simulink model "gm_uz_endat_interface_2023a"  (R2023a)
settings: Solver=FixedStepDiscrete  StartTime=0.0  StopTime=1.3e-3  RelTol=1e-3
undefined symbols (not defined in the file or in its folder): binary_or_gray, bit_sum, delay_first_clk_on_off, endat_clk_divider, endat_encoder_bit_width_multi_turn, endat_encoder_bit_width_single_turn, endat_encoder_number_of_CRC_bits, f_ADC, f_clock, PLL, t_ADC, t_clock
libraries: hdlmdlgenlib x127, simulink x35, hdlsllib x24, simulink_extras x12
(part 3 of 4)

== system gm_uz_endat_interface_2023a/uz_endat_interface/serial_communication/sample_serial_endat_data ==
  note: sample at falling edges of clk
  note: bitset and bit clear
  endat_clk : Inport  OutDataTypeStr=boolean  PortDimensions=1  SampleTime=1e-08
  endat_data : Inport  Port=2  OutDataTypeStr=boolean  PortDimensions=1  SampleTime=1e-08
  sampling_delay_clk_ticks : Inport  Port=3  OutDataTypeStr=uint32  PortDimensions=1  SampleTime=1e-08
  position_sampling_condition_valid : Inport  Port=4  OutDataTypeStr=boolean  PortDimensions=1  SampleTime=1e-08
  Bitwise OR : simulink/Logic and Bit Operations/Bitwise Operator  logicop=OR  UseBitMask=off  NumInputPorts=2  BitMask=double(0)  BitMaskRealWorld=Real World Value
  Bitwise Operator : simulink/Logic and Bit Operations/Bitwise Operator  logicop=AND  UseBitMask=off  NumInputPorts=2  BitMask=double(0)  BitMaskRealWorld=Real World Value
  Bitwise Operator1 : simulink/Logic and Bit Operations/Bitwise Operator  logicop=NOT  UseBitMask=off  BitMask=double(0)  BitMaskRealWorld=Real World Value
  Constant : Constant  Value=0  OutDataTypeStr=boolean  SampleTime=1e-08
  Constant2 : Constant  Value="fi(0,0,64,0,\"hex\",\"0000000000000001\")"  OutDataTypeStr=fixdt(0, 64, 0)  SampleTime=1e-08
  Constant3 : Constant  OutDataTypeStr=boolean  SampleTime=1e-08
  Constant4 : Constant  Value="fi(0,0,64,0,\"hex\",\"0000000000000000\")"  OutDataTypeStr=fixdt(0, 64, 0)  SampleTime=1e-08
  Delay : Delay  DelayLength=double(1)  InitialCondition=0  SampleTime=1e-08
  Delay2 : Delay  DelayLength=double(1)  InitialCondition=0  SampleTime=1e-08
  Detect Rise Positive1 : simulink/Logic and Bit Operations/Detect Rise Positive  vinit=0  OutDataTypeStr=boolean
  Detect Rise Positive2 : simulink/Logic and Bit Operations/Detect Rise Positive  vinit=0  OutDataTypeStr=boolean
  HDL Counter1 : hdlsllib/Sources/HDL Counter  CountType=Free running  CountInit=0  CountStep=1  CountMax=0  CountFromType=Initial value  CountFrom=0  CountResetPort=on  CountLoadPort=off  CountEnbPort=on  CountDirPort=off  CountHitOutputPort=off  CountDataType=Unsigned  CountWordLen=6  CountFracLen=0  CountSampTime=1
  NOT : Logic  Operator=NOT  Inputs=1  AllPortsSameDT=off  OutDataTypeStr=boolean  SampleTime=1e-08
  Relational Operator1 : RelationalOperator  Operator===  OutDataTypeStr=boolean  SampleTime=1e-08  InputSameDT=off
  Relational Operator2 : RelationalOperator  Operator===  OutDataTypeStr=boolean  SampleTime=1e-08  InputSameDT=off
  Sample and Hold1 : Subsystem  mask(Sample and Hold){ic=double(0), Ts=double(1e-08)}
      mask prompts: ic "Initial condition:"; Ts "Sample time:"
      mask help:
      | Sample and hold input signal.
      |
      | The output follows input 1 (In) as long as input 2 (S) is TRUE (1). The output is held when input 2 becomes FALSE (0).
      mask init:
      | Ts = double(1e-08);
      | WantBlockChoice = 'Discrete';
      | block = 'uz_endat_interface_2023a/uz_endat_interface/serial_communication/sample_serial_endat_data/Sample and\nHold1';
      | ic = double(0);
      mask Help: helpview(psbhelp);
      mask Display: disp('S/H')
  Switch : Switch  Criteria=u2 > Threshold  Threshold=double(0)  OutDataTypeStr=boolean  SampleTime=1e-08  SaturateOnIntegerOverflow=off  InputSameDT=off
  Switch1 : Switch  Criteria=u2 > Threshold  Threshold=double(0)  OutDataTypeStr=fixdt(0, 64, 0)  SampleTime=1e-08  SaturateOnIntegerOverflow=off  InputSameDT=off
  Switch3 : Switch  Criteria=u2 > Threshold  Threshold=double(0)  OutDataTypeStr=fixdt(0, 64, 0)  SampleTime=1e-08  SaturateOnIntegerOverflow=off  InputSameDT=off
  Variable Integer Delay : simulink/Discrete/Tapped Delay  vinit=0  samptime=-1  NumDelays=double(100)  DelayOrder=Newest  includeCurrent=on
  multiportswitch : MultiPortSwitch  DataPortOrder=Zero-based contiguous  Inputs=1  DiagnosticForDefault=None  zeroidx=on  SampleTime=1e-08  SaturateOnIntegerOverflow=off  InputSameDT=off
  saturate : Saturate  UpperLimit=double(100)  LowerLimit=double(0)  SampleTime=1e-08  OutDataTypeStr=uint32
  shift arithmetic : ArithShift  BitShiftNumberSource=Input port  BitShiftDirection=Left
      settings: InputPortMap=u0,p1
  endat_data_raw : Outport  OutDataTypeStr=uint64  SampleTime=1e-08
  endat_data_SH : Outport  Port=2  SampleTime=1e-08
  wires:
  Bitwise Operator1/1 -> Bitwise Operator/1
  Constant/1 -> Switch/3
  Constant2/1 -> shift arithmetic/1
  Constant3/1 -> Relational Operator1/2
  Constant4/1 -> Relational Operator2/2
  Detect Rise Positive1/1 -> HDL Counter1/1
  Detect Rise Positive2/1 -> Switch/1
  HDL Counter1/1 -> shift arithmetic/2, Relational Operator2/1
  NOT/1 -> Detect Rise Positive2/1
  Relational Operator1/1 -> Switch1/2
  Relational Operator2/1 -> Switch3/2
  Sample and Hold1/1("   ") -> Relational Operator1/1, endat_data_SH/1
  shift arithmetic/1 -> Bitwise Operator1/1, Bitwise OR/1
  Switch/1 -> Variable Integer Delay/1
  Switch1/1 -> Delay/1, Switch3/1
  Switch3/1 -> endat_data_raw/1, Delay2/1
  multiportswitch/1 -> Sample and Hold1/2(S), HDL Counter1/2
  Variable Integer Delay/1 -> multiportswitch/2
  saturate/1 -> multiportswitch/1
  endat_clk/1 -> NOT/1
  endat_data/1 -> Sample and Hold1/1(In)
  sampling_delay_clk_ticks/1 -> saturate/1
  position_sampling_condition_valid/1 -> Switch/2, Detect Rise Positive1/1
  Delay2/1 -> Switch3/3
  Delay/1 -> Bitwise Operator/2
  Bitwise Operator/1 -> Switch1/3, Bitwise OR/2
  Bitwise OR/1 -> Switch1/1

== system gm_uz_endat_interface_2023a/uz_endat_interface/serial_communication/ssi_clock_generator ==
  endat_clk_divider : Inport  OutDataTypeStr=uint32  PortDimensions=1  SampleTime=1e-08
  endat_clk_reset : Inport  Port=2  OutDataTypeStr=boolean  PortDimensions=1  SampleTime=1e-08
  endat_clk_enb : Inport  Port=3  OutDataTypeStr=boolean  PortDimensions=1  SampleTime=1e-08
  AND : Logic  AllPortsSameDT=off  OutDataTypeStr=boolean  SampleTime=1e-08
  AND1 : Logic  AllPortsSameDT=off  OutDataTypeStr=boolean  SampleTime=1e-08
  Constant : Constant  OutDataTypeStr=uint16  SampleTime=1e-08
  Data Type Conversion : DataTypeConversion  OutDataTypeStr=uint16  SampleTime=1e-08  SaturateOnIntegerOverflow=off  RndMeth=Floor
  Delay : Delay  DelayLength=double(1)  InitialCondition=0  SampleTime=1e-08
  Delay1 : Delay  DelayLength=double(1)  InitialCondition=0  SampleTime=1e-08
  Detect Rise Positive1 : simulink/Logic and Bit Operations/Detect Rise Positive  vinit=0  OutDataTypeStr=boolean
  OR : Logic  Operator=OR  AllPortsSameDT=off  OutDataTypeStr=boolean  SampleTime=1e-08
  Relational Operator : RelationalOperator  OutDataTypeStr=boolean  SampleTime=1e-08  InputSameDT=off
  S-R Flip-Flop1 : simulink_extras/Flip Flops/S-R Flip-Flop  initial_condition=0
  Sum : Sum  Inputs=+-  AccumDataTypeStr=uint16  OutDataTypeStr=uint16  SampleTime=1e-08
  base_counter : hdlsllib/Sources/HDL Counter  CountType=Free running  CountInit=0  CountStep=1  CountMax=199  CountFromType=Initial value  CountFrom=0  CountResetPort=on  CountLoadPort=off  CountEnbPort=on  CountDirPort=off  CountHitOutputPort=off  CountDataType=Unsigned  CountWordLen=16  CountFracLen=0  CountSampTime=1
  endat_clk : Outport  SampleTime=1e-08
  wires:
  Constant/1 -> Sum/2
  Data Type Conversion/1 -> Sum/1
  Detect Rise Positive1/1 -> AND1/2, AND/1
  S-R Flip-Flop1/1 -> endat_clk/1, Delay/1
  Sum/1 -> Relational Operator/2
  base_counter/1 -> Detect Rise Positive1/1, Relational Operator/1
  endat_clk_divider/1 -> Data Type Conversion/1
  endat_clk_reset/1 -> OR/2
  endat_clk_enb/1 -> base_counter/2
  Delay/1 -> AND/2
  AND1/1 -> S-R Flip-Flop1/1
  Delay1/1 -> AND1/1
  S-R Flip-Flop1/2 -> Delay1/1
  OR/1 -> S-R Flip-Flop1/2
  AND/1 -> OR/1
  Relational Operator/1 -> base_counter/1

== system gm_uz_endat_interface_2023a/uz_endat_interface/set_offset_to_raw_position_and_wrap/floor_div_pow2 ==
  dividend : Inport  OutDataTypeStr=fixdt(1, 64, 0)  PortDimensions=1  SampleTime=1e-08
  divisor_power_of_two_bits : Inport  Port=2  OutDataTypeStr=uint32  PortDimensions=1  SampleTime=1e-08
  AND2 : Logic  AllPortsSameDT=off  OutDataTypeStr=boolean  SampleTime=1e-08
  Bitwise AND6 : simulink/Logic and Bit Operations/Bitwise Operator  logicop=AND  UseBitMask=off  NumInputPorts=2  BitMask=double(0)  BitMaskRealWorld=Real World Value
  Constant : Constant  Value="fi(0,1,64,0,\"hex\",\"0000000000000000\")"  OutDataTypeStr=fixdt(1, 64, 0)  SampleTime=1e-08
  Relational Operator : RelationalOperator  Operator=<  OutDataTypeStr=boolean  SampleTime=1e-08  InputSameDT=off
  Relational Operator1 : RelationalOperator  Operator=~=  OutDataTypeStr=boolean  SampleTime=1e-08  InputSameDT=off
  Sum10 : Sum  Inputs=+-  AccumDataTypeStr=fixdt(1, 65, 0)  OutDataTypeStr=fixdt(1, 64, 0)  SampleTime=1e-08
  Sum9 : Sum  Inputs=+-  AccumDataTypeStr=fixdt(1, 65, 0)  OutDataTypeStr=fixdt(1, 64, 0)  SampleTime=1e-08
  Switch : Switch  Criteria=u2 > Threshold  Threshold=double(0)  OutDataTypeStr=fixdt(1, 64, 0)  SampleTime=1e-08  SaturateOnIntegerOverflow=off  InputSameDT=off
  const4 : Constant  Value="fi(0,1,64,0,\"hex\",\"0000000000000001\")"  OutDataTypeStr=fixdt(1, 64, 0)  SampleTime=1e-08
  shift arithmetic4 : ArithShift  BitShiftNumberSource=Input port  BitShiftDirection=Right
      settings: InputPortMap=u0,p1
  shift arithmetic5 : ArithShift  BitShiftNumberSource=Input port  BitShiftDirection=Left
      settings: InputPortMap=u0,p1
  quotient : Outport  SampleTime=1e-08
  wires:
  AND2/1 -> Switch/2
  Bitwise AND6/1 -> Relational Operator1/1
  Constant/1 -> Relational Operator1/2, Relational Operator/2
  Relational Operator/1 -> AND2/1
  Relational Operator1/1 -> AND2/2
  shift arithmetic4/1 -> Switch/3, Sum10/1
  shift arithmetic5/1 -> Sum9/1
  Sum10/1 -> Switch/1
  Sum9/1 -> Bitwise AND6/2
  Switch/1 -> quotient/1
  const4/1 -> Sum9/2, Sum10/2, shift arithmetic5/1
  dividend/1 -> shift arithmetic4/1, Relational Operator/1, Bitwise AND6/1
  divisor_power_of_two_bits/1 -> shift arithmetic5/2, shift arithmetic4/2

== system gm_uz_endat_interface_2023a/uz_endat_interface/wrap_2pi/fixed_point_floor ==
  x : Inport  OutDataTypeStr=fixdt(0, 27, 24)  PortDimensions=1  SampleTime=1e-08
  fixed_point_floor : MATLAB Function  TreatAsAtomicUnit=on
  y : Outport  SampleTime=1e-08  VectorParamsAs1DForOutWhenUnconnected=off
  wires:
  fixed_point_floor/1(y) -> y/1
  x/1 -> fixed_point_floor/1(x)

== system gm_uz_endat_interface_2023a/uz_endat_interface/position_to_speed_pll/Sine HDL Optimized/sincos hdl ==
  In1 : Inport  OutDataTypeStr=fixdt(1, 27, 20)  SampleTime=1e-08
  cos_hdl : Subsystem  mask{NumDataPoints=double(256), TableDataTypeStr=fixdt(0,26,20), SimulateLUTROMDelay=Off}
      mask prompts: NumDataPoints "HDLShared:hdlshared:CosineHDL_Npts"; TableDataTypeStr "Simulink:blkprm_prompts:TABLE_UNIFIEDDATATYPE"; SimulateLUTROMDelay "HDLShared:hdlshared:CosineHDL_SimulateLUTDelay"
      mask Display:
      | port_label('input',1,'u')
      | port_label('output',1,'cos(2*pi*u)')
      | xpos = 0.35;
      | yoffset = 0.5;
      | if ( SimulateLUTROMDelay )
      |   text(xpos,yoffset,'HDL (Z^{-1})','texmode','on')
      | else
      |    text(xpos,yoffset,'HDL')
      | end
  sin_hdl : Subsystem  mask{NumDataPoints=double(256), TableDataTypeStr=fixdt(0,26,20), SimulateLUTROMDelay=Off}
      mask prompts: NumDataPoints "HDLShared:hdlshared:CosineHDL_Npts"; TableDataTypeStr "Simulink:blkprm_prompts:TABLE_UNIFIEDDATATYPE"; SimulateLUTROMDelay "HDLShared:hdlshared:CosineHDL_SimulateLUTDelay"
      mask Display:
      | port_label('input',1,'u')
      | port_label('output',1,'sin(2*pi*u)')
      | xpos = 0.35;
      | yoffset = 0.5;
      | if ( SimulateLUTROMDelay )
      |   text(xpos,yoffset,'HDL (Z^{-1})','texmode','on')
      | else
      |    text(xpos,yoffset,'HDL')
      | end
  Out1 : Outport  SampleTime=1e-08  InitialOutput=0
  Out2 : Outport  Port=2  SampleTime=1e-08  InitialOutput=0
  wires:
  cos_hdl/1(x) -> Out2/1
  sin_hdl/1(y) -> Out1/1
  In1/1 -> cos_hdl/1(In1), sin_hdl/1(In1)

== system gm_uz_endat_interface_2023a/uz_endat_interface/position_to_speed_pll/Sine HDL Optimized1/sincos hdl ==
  In1 : Inport  OutDataTypeStr=fixdt(1, 27, 20)  SampleTime=1e-08
  cos_hdl : Subsystem  mask{NumDataPoints=double(256), TableDataTypeStr=fixdt(0,26,20), SimulateLUTROMDelay=Off}
      mask prompts: NumDataPoints "HDLShared:hdlshared:CosineHDL_Npts"; TableDataTypeStr "Simulink:blkprm_prompts:TABLE_UNIFIEDDATATYPE"; SimulateLUTROMDelay "HDLShared:hdlshared:CosineHDL_SimulateLUTDelay"
      mask Display:
      | port_label('input',1,'u')
      | port_label('output',1,'cos(2*pi*u)')
      | xpos = 0.35;
      | yoffset = 0.5;
      | if ( SimulateLUTROMDelay )
      |   text(xpos,yoffset,'HDL (Z^{-1})','texmode','on')
      | else
      |    text(xpos,yoffset,'HDL')
      | end
  sin_hdl : Subsystem  mask{NumDataPoints=double(256), TableDataTypeStr=fixdt(0,26,20), SimulateLUTROMDelay=Off}
      mask prompts: NumDataPoints "HDLShared:hdlshared:CosineHDL_Npts"; TableDataTypeStr "Simulink:blkprm_prompts:TABLE_UNIFIEDDATATYPE"; SimulateLUTROMDelay "HDLShared:hdlshared:CosineHDL_SimulateLUTDelay"
      mask Display:
      | port_label('input',1,'u')
      | port_label('output',1,'sin(2*pi*u)')
      | xpos = 0.35;
      | yoffset = 0.5;
      | if ( SimulateLUTROMDelay )
      |   text(xpos,yoffset,'HDL (Z^{-1})','texmode','on')
      | else
      |    text(xpos,yoffset,'HDL')
      | end
  Out1 : Outport  SampleTime=1e-08  InitialOutput=0
  Out2 : Outport  Port=2  SampleTime=1e-08  InitialOutput=0
  wires:
  cos_hdl/1(x) -> Out2/1
  sin_hdl/1(y) -> Out1/1
  In1/1 -> cos_hdl/1(In1), sin_hdl/1(In1)

== system gm_uz_endat_interface_2023a/uz_endat_interface/serial_communication/sample_serial_endat_data/Sample and Hold1 ==
  In : Inport  OutDataTypeStr=boolean  SampleTime=1e-08
  S : Inport  Port=2  OutDataTypeStr=boolean  SampleTime=1e-08
  Model : Subsystem
  "   " : Outport  SampleTime=1e-08
  wires:
  Model/1(Out) -> "   "/1
  In/1 -> Model/1(In)
  S/1 -> Model/2(S)

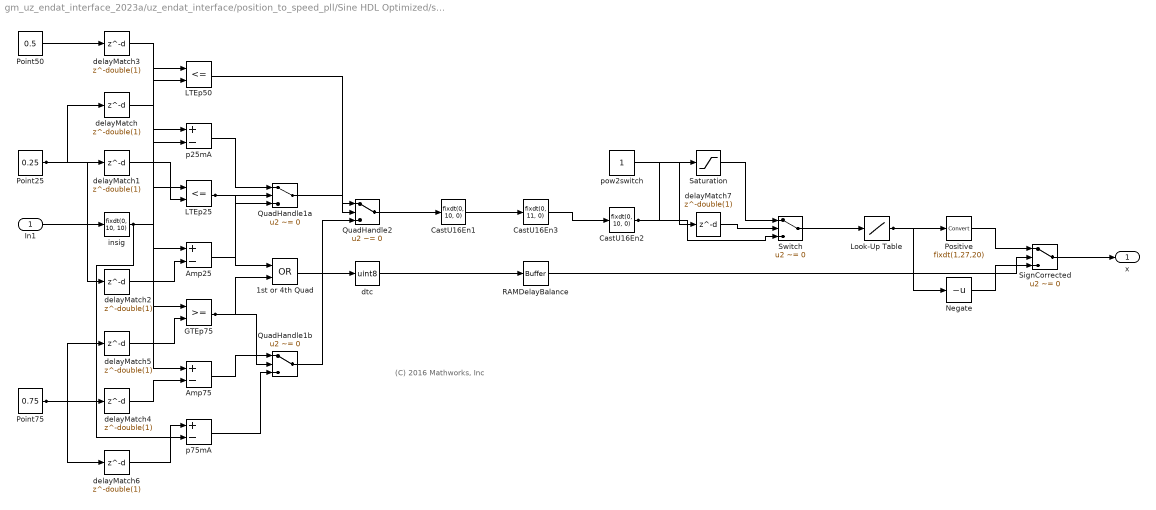
== system gm_uz_endat_interface_2023a/uz_endat_interface/position_to_speed_pll/Sine HDL Optimized/sincos hdl/cos_hdl ==
  note: (C) 2016 Mathworks, Inc
  In1 : Inport  OutDataTypeStr=fixdt(1, 27, 20)  SampleTime=1e-08
  1st or 4th Quad : Logic  Operator=OR  AllPortsSameDT=off  OutDataTypeStr=boolean  SampleTime=1e-08
  Amp25 : Sum  Inputs=+-  AccumDataTypeStr=fixdt(1, 28, 27)  OutDataTypeStr=fixdt(1, 28, 27)  SampleTime=1e-08
  Amp75 : Sum  Inputs=+-  AccumDataTypeStr=fixdt(1, 28, 27)  OutDataTypeStr=fixdt(1, 28, 27)  SampleTime=1e-08
  CastU16En1 : DataTypeConversion  OutDataTypeStr=fixdt(0, 10, 0)  ConvertRealWorld=Stored Integer (SI)  SampleTime=1e-08  SaturateOnIntegerOverflow=off  RndMeth=Floor
  CastU16En2 : DataTypeConversion  OutDataTypeStr=fixdt(0, 10, 0)  ConvertRealWorld=Stored Integer (SI)  SampleTime=1e-08  RndMeth=Floor
  CastU16En3 : DataTypeConversion  OutDataTypeStr=fixdt(0, 11, 0)  SampleTime=1e-08  SaturateOnIntegerOverflow=off  RndMeth=Floor
  GTEp75 : RelationalOperator  OutDataTypeStr=boolean  SampleTime=1e-08  InputSameDT=off
  LTEp25 : RelationalOperator  Operator=<=  OutDataTypeStr=boolean  SampleTime=1e-08  InputSameDT=off
  LTEp50 : RelationalOperator  Operator=<=  OutDataTypeStr=boolean  SampleTime=1e-08  InputSameDT=off
  Look-Up Table : Lookup_n-D  NumberOfTableDimensions=1  BreakpointsForDimension1="fi(\"numerictype\",numerictype(0,10,0),\"fimath\",fimath(\"RoundingMethod\", \"Floor\",\"OverflowAction\", \"Wrap\",\"ProductMode\",\"FullPrecision\",\"SumMode\",\"FullPrecision\"),\"Value\",\"[0 1 2 3 4 5 6 7 8 9 10 11 12 13 14 15 16 17 18 19 20 21 22 23 24 25 26 27 28 29 30 31 32 33 34 35 36 37 38 39 40 41 42 43 44 45 46 47 48 49 50 51 52 53 54 55 56 57 58 59 60 61 62 63 64 65 66 67 68 69 70 71 72 73 74 75 76 77 78 79 80 81 82 83 84 85 86 87 88 89 90 91 92 93 94 95 96 97 98 99 100 101 102 103 104 105 106 107 108 109 110 111 112 113 114 115 116 117 118 119 120 121 122 123 124 125 126 127 128 129 130 131 132 133 134 135 136 137 138 139 140 141 142 143 144 145 146 147 148 149 150 151 152 153 154 155 156 157 158 159 160 161 162 163 164 165 166 167 168 169 170 171 172 173 174 175 176 177 178 179 180 181 182 183 184 185 186 187 188 189 190 191 192 193 194 195 196 197 198 199 200 201 202 203 204 205 206 207 208 209 210 211 212 213 214 215 216 217 218 219 220 221 222 223 224 225 226 227 228 229 230 231 232 233 234 235 236 237 238 239 240 241 242 243 244 245 246 247 248 249 250 251 252 253 254 255]\")"  Table="reshape(fi(\"numerictype\",numerictype(1,27,20),\"fimath\",fimath(\"RoundingMethod\", \"Floor\",\"OverflowAction\", \"Wrap\",\"ProductMode\",\"FullPrecision\",\"SumMode\",\"FullPrecision\"),\"Value\",\"[0;0.0061359405517578125;0.012271881103515625;0.01840686798095703125;0.02454090118408203125;0.03067493438720703125;0.03680706024169921875;0.042938232421875;0.04906749725341796875;0.055194854736328125;0.06132030487060546875;0.06744384765625;0.0735645294189453125;0.07968235015869140625;0.08579730987548828125;0.0919094085693359375;0.0980167388916015625;0.10412120819091796875;0.11022186279296875;0.11631870269775390625;0.12241077423095703125;0.128498077392578125;0.1345806121826171875;0.14065837860107421875;0.1467304229736328125;0.15279674530029296875;0.15885829925537109375;0.164913177490234375;0.17096233367919921875;0.1770038604736328125;0.18303966522216796875;0.18906879425048828125;0.19509029388427734375;0.20110416412353515625;0.207111358642578125;0.2131099700927734375;0.2191009521484375;0.2250843048095703125;0.2310581207275390625;0.23702335357666015625;0.24298000335693359375;0.248928070068359375;0.2548656463623046875;0.2607936859130859375;0.26671314239501953125;0.27262115478515625;0.27851963043212890625;0.28440761566162109375;0.2902851104736328125;0.29615116119384765625;0.302005767822265625;0.307849884033203125;0.31368160247802734375;0.3195018768310546875;0.32531070709228515625;0.3311061859130859375;0.33689022064208984375;0.3426609039306640625;0.34841823577880859375;0.35416316986083984375;0.35989475250244140625;0.36561298370361328125;0.3713169097900390625;0.37700748443603515625;0.38268375396728515625;0.38834476470947265625;0.39399242401123046875;0.399623870849609375;0.4052410125732421875;0.4108428955078125;0.4164295196533203125;0.42199993133544921875;0.427555084228515625;0.433094024658203125;0.4386157989501953125;0.444122314453125;0.449611663818359375;0.4550838470458984375;0.4605388641357421875;0.465976715087890625;0.47139644622802734375;0.47679901123046875;0.4821834564208984375;0.48754978179931640625;0.49289798736572265625;0.4982280731201171875;0.5035381317138671875;0.50883007049560546875;0.514102935791015625;0.51935577392578125;0.52458953857421875;0.52980327606201171875;0.5349979400634765625;0.54017162322998046875;0.54532527923583984375;0.55045795440673828125;0.5555706024169921875;0.56066131591796875;0.56573200225830078125;0.57078075408935546875;0.57580852508544921875;0.580814361572265625;0.5857982635498046875;0.59075927734375;0.595699310302734375;0.600616455078125;0.605510711669921875;0.61038303375244140625;0.61523151397705078125;0.62005710601806640625;0.62485980987548828125;0.629638671875;0.6343936920166015625;0.63912487030029296875;0.6438312530517578125;0.64851474761962890625;0.65317249298095703125;0.657806396484375;0.66241550445556640625;0.66699981689453125;0.67155933380126953125;0.67609310150146484375;0.6806011199951171875;0.6850833892822265625;0.689540863037109375;0.6939716339111328125;0.69837665557861328125;0.702754974365234375;0.70710659027099609375;0.71143245697021484375;0.7157306671142578125;0.72000217437744140625;0.724246978759765625;0.7284641265869140625;0.732654571533203125;0.73681640625;0.7409515380859375;0.7450580596923828125;0.7491359710693359375;0.7531871795654296875;0.75720882415771484375;0.76120281219482421875;0.765167236328125;0.76910305023193359375;0.77301025390625;0.77688884735107421875;0.7807369232177734375;0.78455638885498046875;0.78834629058837890625;0.79210662841796875;0.79583644866943359375;0.79953765869140625;0.8032073974609375;0.80684757232666015625;0.8104572296142578125;0.81403636932373046875;0.817584991455078125;0.821102142333984375;0.82458972930908203125;0.828044891357421875;0.83146953582763671875;0.83486270904541015625;0.8382244110107421875;0.8415546417236328125;0.84485340118408203125;0.84812068939208984375;0.85135555267333984375;0.85455799102783203125;0.8577289581298828125;0.860866546630859375;0.86397266387939453125;0.867046356201171875;0.870086669921875;0.8730945587158203125;0.8760700225830078125;0.87901210784912109375;0.88192081451416015625;0.88479709625244140625;0.8876399993896484375;0.89044857025146484375;0.8932247161865234375;0.89596652984619140625;0.89867401123046875 ...(+1615 chars)]\"), [1  256])"  InterpMethod=Flat  ExtrapMethod=Clip  DiagnosticForOutOfRangeInput=Error  SampleTime=1e-08  OutDataTypeStr=fixdt(1, 27, 20)
  Negate : UnaryMinus  SampleTime=1e-08
  Point25 : Constant  Value=0.25  OutDataTypeStr=fixdt(0, 27, 27)  SampleTime=1e-08
  Point50 : Constant  Value=0.5  OutDataTypeStr=fixdt(0, 27, 27)  SampleTime=1e-08
  Point75 : Constant  Value=0.75  OutDataTypeStr=fixdt(0, 27, 27)  SampleTime=1e-08
  Positive : DataTypeConversion  OutDataTypeStr=fixdt(1,27,20)
  QuadHandle1a : Switch  Criteria=u2 ~= 0  Threshold=double(0)  OutDataTypeStr=fixdt(1, 28, 27)  SampleTime=1e-08  SaturateOnIntegerOverflow=off  InputSameDT=off
  QuadHandle1b : Switch  Criteria=u2 ~= 0  Threshold=double(0)  OutDataTypeStr=fixdt(1, 28, 27)  SampleTime=1e-08  SaturateOnIntegerOverflow=off  InputSameDT=off
  QuadHandle2 : Switch  Criteria=u2 ~= 0  Threshold=double(0)  OutDataTypeStr=fixdt(0, 10, 10)  SampleTime=1e-08  InputSameDT=off
  RAMDelayBalance : hdlmdlgenlib/Buffer
  Saturation : Saturate  UpperLimit="fi(0,0,10,0,\"hex\",\"0ff\")"  LowerLimit="fi(0,0,10,0,\"hex\",\"000\")"  SampleTime=1e-08  OutDataTypeStr=fixdt(0, 10, 0)
  SignCorrected : Switch  Criteria=u2 ~= 0  Threshold=double(0)  OutDataTypeStr=fixdt(1, 27, 20)  SampleTime=1e-08  SaturateOnIntegerOverflow=off  InputSameDT=off
  Switch : Switch  Criteria=u2 ~= 0  Threshold=double(0)  OutDataTypeStr=fixdt(0, 10, 0)  SampleTime=1e-08  SaturateOnIntegerOverflow=off  InputSameDT=off
  delayMatch{,1..7} (8 alike) : Delay  DelayLength=double(1)  InitialCondition=0
  dtc : DataTypeConversion  OutDataTypeStr=uint8  ConvertRealWorld=Stored Integer (SI)  SampleTime=1e-08  SaturateOnIntegerOverflow=off  RndMeth=Floor
  insig : DataTypeConversion  OutDataTypeStr=fixdt(0, 10, 10)  SampleTime=1e-08  SaturateOnIntegerOverflow=off  RndMeth=Floor
  p25mA : Sum  Inputs=+-  AccumDataTypeStr=fixdt(1, 28, 27)  OutDataTypeStr=fixdt(1, 28, 27)  SampleTime=1e-08
  p75mA : Sum  Inputs=+-  AccumDataTypeStr=fixdt(1, 28, 27)  OutDataTypeStr=fixdt(1, 28, 27)  SampleTime=1e-08
  pow2switch : Constant  OutDataTypeStr=boolean  SampleTime=1e-08
  x : Outport  SampleTime=1e-08  InitialOutput=0
  wires:
  dtc/1 -> RAMDelayBalance/1
  Amp25/1 -> QuadHandle1a/3
  Amp75/1 -> QuadHandle1b/1
  CastU16En1/1 -> CastU16En3/1
  CastU16En2/1 -> Switch/3, Saturation/1
  CastU16En3/1 -> CastU16En2/1
  GTEp75/1 -> QuadHandle1b/2, 1st or 4th Quad/2
  LTEp25/1 -> QuadHandle1a/2, 1st or 4th Quad/1
  LTEp50/1 -> QuadHandle2/2
  Look-Up Table/1 -> Positive/1, Negate/1
  Negate/1 -> SignCorrected/3
  delayMatch/1 -> p25mA/1
  delayMatch3/1 -> LTEp50/2
  delayMatch4/1 -> Amp75/2
  Positive/1 -> SignCorrected/1
  QuadHandle1a/1 -> QuadHandle2/1
  QuadHandle1b/1 -> QuadHandle2/3
  QuadHandle2/1 -> CastU16En1/1
  RAMDelayBalance/1 -> SignCorrected/2
  Saturation/1 -> Switch/1
  SignCorrected/1 -> x/1
  Switch/1 -> Look-Up Table/1
  insig/1 -> p75mA/2, p25mA/2, LTEp50/1, LTEp25/1, GTEp75/1, Amp75/1, Amp25/1
  p25mA/1 -> QuadHandle1a/1
  p75mA/1 -> QuadHandle1b/3
  delayMatch7/1 -> Switch/2
  1st or 4th Quad/1 -> dtc/1
  In1/1 -> insig/1
  delayMatch1/1 -> LTEp25/2
  delayMatch2/1 -> Amp25/2
  Point25/1 -> delayMatch2/1, delayMatch1/1, delayMatch/1
  Point50/1 -> delayMatch3/1
  delayMatch5/1 -> GTEp75/2
  delayMatch6/1 -> p75mA/1
  Point75/1 -> delayMatch6/1, delayMatch5/1, delayMatch4/1
  pow2switch/1 -> delayMatch7/1

== system gm_uz_endat_interface_2023a/uz_endat_interface/position_to_speed_pll/Sine HDL Optimized/sincos hdl/sin_hdl ==
  note: (C) 2016 Mathworks, Inc
  In1 : Inport  OutDataTypeStr=fixdt(1, 27, 20)  SampleTime=1e-08
  Amp50 : Sum  Inputs=+-  AccumDataTypeStr=fixdt(1, 28, 27)  OutDataTypeStr=fixdt(1, 28, 27)  SampleTime=1e-08
  CastU16En2 : DataTypeConversion  OutDataTypeStr=fixdt(0, 10, 0)  ConvertRealWorld=Stored Integer (SI)  SampleTime=1e-08  SaturateOnIntegerOverflow=off  RndMeth=Floor
  CastU16En3 : DataTypeConversion  OutDataTypeStr=fixdt(0, 10, 0)  ConvertRealWorld=Stored Integer (SI)  SampleTime=1e-08  RndMeth=Floor
  CastU16En4 : DataTypeConversion  OutDataTypeStr=fixdt(0, 11, 0)  SampleTime=1e-08  SaturateOnIntegerOverflow=off  RndMeth=Floor
  LTEp25 : RelationalOperator  Operator=<=  OutDataTypeStr=boolean  SampleTime=1e-08  InputSameDT=off
  LTEp50 : RelationalOperator  Operator=<=  OutDataTypeStr=boolean  SampleTime=1e-08  InputSameDT=off
  Look-Up Table : Lookup_n-D  NumberOfTableDimensions=1  BreakpointsForDimension1="fi(\"numerictype\",numerictype(0,10,0),\"fimath\",fimath(\"RoundingMethod\", \"Floor\",\"OverflowAction\", \"Wrap\",\"ProductMode\",\"FullPrecision\",\"SumMode\",\"FullPrecision\"),\"Value\",\"[0 1 2 3 4 5 6 7 8 9 10 11 12 13 14 15 16 17 18 19 20 21 22 23 24 25 26 27 28 29 30 31 32 33 34 35 36 37 38 39 40 41 42 43 44 45 46 47 48 49 50 51 52 53 54 55 56 57 58 59 60 61 62 63 64 65 66 67 68 69 70 71 72 73 74 75 76 77 78 79 80 81 82 83 84 85 86 87 88 89 90 91 92 93 94 95 96 97 98 99 100 101 102 103 104 105 106 107 108 109 110 111 112 113 114 115 116 117 118 119 120 121 122 123 124 125 126 127 128 129 130 131 132 133 134 135 136 137 138 139 140 141 142 143 144 145 146 147 148 149 150 151 152 153 154 155 156 157 158 159 160 161 162 163 164 165 166 167 168 169 170 171 172 173 174 175 176 177 178 179 180 181 182 183 184 185 186 187 188 189 190 191 192 193 194 195 196 197 198 199 200 201 202 203 204 205 206 207 208 209 210 211 212 213 214 215 216 217 218 219 220 221 222 223 224 225 226 227 228 229 230 231 232 233 234 235 236 237 238 239 240 241 242 243 244 245 246 247 248 249 250 251 252 253 254 255]\")"  Table="reshape(fi(\"numerictype\",numerictype(1,27,20),\"fimath\",fimath(\"RoundingMethod\", \"Floor\",\"OverflowAction\", \"Wrap\",\"ProductMode\",\"FullPrecision\",\"SumMode\",\"FullPrecision\"),\"Value\",\"[0;0.0061359405517578125;0.012271881103515625;0.01840686798095703125;0.02454090118408203125;0.03067493438720703125;0.03680706024169921875;0.042938232421875;0.04906749725341796875;0.055194854736328125;0.06132030487060546875;0.06744384765625;0.0735645294189453125;0.07968235015869140625;0.08579730987548828125;0.0919094085693359375;0.0980167388916015625;0.10412120819091796875;0.11022186279296875;0.11631870269775390625;0.12241077423095703125;0.128498077392578125;0.1345806121826171875;0.14065837860107421875;0.1467304229736328125;0.15279674530029296875;0.15885829925537109375;0.164913177490234375;0.17096233367919921875;0.1770038604736328125;0.18303966522216796875;0.18906879425048828125;0.19509029388427734375;0.20110416412353515625;0.207111358642578125;0.2131099700927734375;0.2191009521484375;0.2250843048095703125;0.2310581207275390625;0.23702335357666015625;0.24298000335693359375;0.248928070068359375;0.2548656463623046875;0.2607936859130859375;0.26671314239501953125;0.27262115478515625;0.27851963043212890625;0.28440761566162109375;0.2902851104736328125;0.29615116119384765625;0.302005767822265625;0.307849884033203125;0.31368160247802734375;0.3195018768310546875;0.32531070709228515625;0.3311061859130859375;0.33689022064208984375;0.3426609039306640625;0.34841823577880859375;0.35416316986083984375;0.35989475250244140625;0.36561298370361328125;0.3713169097900390625;0.37700748443603515625;0.38268375396728515625;0.38834476470947265625;0.39399242401123046875;0.399623870849609375;0.4052410125732421875;0.4108428955078125;0.4164295196533203125;0.42199993133544921875;0.427555084228515625;0.433094024658203125;0.4386157989501953125;0.444122314453125;0.449611663818359375;0.4550838470458984375;0.4605388641357421875;0.465976715087890625;0.47139644622802734375;0.47679901123046875;0.4821834564208984375;0.48754978179931640625;0.49289798736572265625;0.4982280731201171875;0.5035381317138671875;0.50883007049560546875;0.514102935791015625;0.51935577392578125;0.52458953857421875;0.52980327606201171875;0.5349979400634765625;0.54017162322998046875;0.54532527923583984375;0.55045795440673828125;0.5555706024169921875;0.56066131591796875;0.56573200225830078125;0.57078075408935546875;0.57580852508544921875;0.580814361572265625;0.5857982635498046875;0.59075927734375;0.595699310302734375;0.600616455078125;0.605510711669921875;0.61038303375244140625;0.61523151397705078125;0.62005710601806640625;0.62485980987548828125;0.629638671875;0.6343936920166015625;0.63912487030029296875;0.6438312530517578125;0.64851474761962890625;0.65317249298095703125;0.657806396484375;0.66241550445556640625;0.66699981689453125;0.67155933380126953125;0.67609310150146484375;0.6806011199951171875;0.6850833892822265625;0.689540863037109375;0.6939716339111328125;0.69837665557861328125;0.702754974365234375;0.70710659027099609375;0.71143245697021484375;0.7157306671142578125;0.72000217437744140625;0.724246978759765625;0.7284641265869140625;0.732654571533203125;0.73681640625;0.7409515380859375;0.7450580596923828125;0.7491359710693359375;0.7531871795654296875;0.75720882415771484375;0.76120281219482421875;0.765167236328125;0.76910305023193359375;0.77301025390625;0.77688884735107421875;0.7807369232177734375;0.78455638885498046875;0.78834629058837890625;0.79210662841796875;0.79583644866943359375;0.79953765869140625;0.8032073974609375;0.80684757232666015625;0.8104572296142578125;0.81403636932373046875;0.817584991455078125;0.821102142333984375;0.82458972930908203125;0.828044891357421875;0.83146953582763671875;0.83486270904541015625;0.8382244110107421875;0.8415546417236328125;0.84485340118408203125;0.84812068939208984375;0.85135555267333984375;0.85455799102783203125;0.8577289581298828125;0.860866546630859375;0.86397266387939453125;0.867046356201171875;0.870086669921875;0.8730945587158203125;0.8760700225830078125;0.87901210784912109375;0.88192081451416015625;0.88479709625244140625;0.8876399993896484375;0.89044857025146484375;0.8932247161865234375;0.89596652984619140625;0.89867401123046875 ...(+1615 chars)]\"), [1  256])"  InterpMethod=Flat  ExtrapMethod=Clip  DiagnosticForOutOfRangeInput=Error  SampleTime=1e-08  OutDataTypeStr=fixdt(1, 27, 20)
  Negate : UnaryMinus  SampleTime=1e-08
  Point25 : Constant  Value=0.25  OutDataTypeStr=fixdt(0, 27, 27)  SampleTime=1e-08
  Point50 : Constant  Value=0.5  OutDataTypeStr=fixdt(0, 27, 27)  SampleTime=1e-08
  Positive : DataTypeConversion  OutDataTypeStr=fixdt(1,27,20)
  QuadHandle1 : Switch  Criteria=u2 ~= 0  Threshold=double(0)  OutDataTypeStr=fixdt(1, 28, 27)  SampleTime=1e-08  SaturateOnIntegerOverflow=off  InputSameDT=off
  QuadHandle2 : Switch  Criteria=u2 ~= 0  Threshold=double(0)  OutDataTypeStr=fixdt(0, 10, 10)  SampleTime=1e-08  SaturateOnIntegerOverflow=off  InputSameDT=off
  RAMDelayBalance : hdlmdlgenlib/Buffer
  Saturation : Saturate  UpperLimit="fi(0,0,10,0,\"hex\",\"0ff\")"  LowerLimit="fi(0,0,10,0,\"hex\",\"000\")"  SampleTime=1e-08  OutDataTypeStr=fixdt(0, 10, 0)
  SignCorrected : Switch  Criteria=u2 ~= 0  Threshold=double(0)  OutDataTypeStr=fixdt(1, 27, 20)  SampleTime=1e-08  SaturateOnIntegerOverflow=off  InputSameDT=off
  Switch : Switch  Criteria=u2 ~= 0  Threshold=double(0)  OutDataTypeStr=fixdt(0, 10, 0)  SampleTime=1e-08  SaturateOnIntegerOverflow=off  InputSameDT=off
  delayMatch{,1..4} (5 alike) : Delay  DelayLength=double(1)  InitialCondition=0
  insig : DataTypeConversion  OutDataTypeStr=fixdt(0, 10, 10)  SampleTime=1e-08  SaturateOnIntegerOverflow=off  RndMeth=Floor
  p50mA : Sum  Inputs=+-  AccumDataTypeStr=fixdt(1, 29, 27)  OutDataTypeStr=fixdt(1, 29, 27)  SampleTime=1e-08
  pow2switch : Constant  OutDataTypeStr=boolean  SampleTime=1e-08
  y : Outport  SampleTime=1e-08  InitialOutput=0
  wires:
  Amp50/1 -> QuadHandle1/3
  CastU16En2/1 -> CastU16En4/1
  CastU16En3/1 -> Switch/3, Saturation/1
  CastU16En4/1 -> CastU16En3/1
  LTEp25/1 -> QuadHandle2/2
  LTEp50/1 -> QuadHandle1/2, RAMDelayBalance/1
  Look-Up Table/1 -> Positive/1, Negate/1
  Negate/1 -> SignCorrected/3
  delayMatch2/1 -> LTEp25/2
  delayMatch/1 -> LTEp50/2
  Positive/1 -> SignCorrected/1
  QuadHandle1/1 -> p50mA/2, QuadHandle2/1, LTEp25/1
  QuadHandle2/1 -> CastU16En2/1
  RAMDelayBalance/1 -> SignCorrected/2
  Saturation/1 -> Switch/1
  SignCorrected/1 -> y/1
  Switch/1 -> Look-Up Table/1
  insig/1 -> QuadHandle1/1, LTEp50/1, Amp50/1
  p50mA/1 -> QuadHandle2/3
  delayMatch4/1 -> Switch/2
  In1/1 -> insig/1
  delayMatch1/1 -> Amp50/2
  delayMatch3/1 -> p50mA/1
  Point25/1 -> delayMatch2/1
  Point50/1 -> delayMatch3/1, delayMatch1/1, delayMatch/1
  pow2switch/1 -> delayMatch4/1

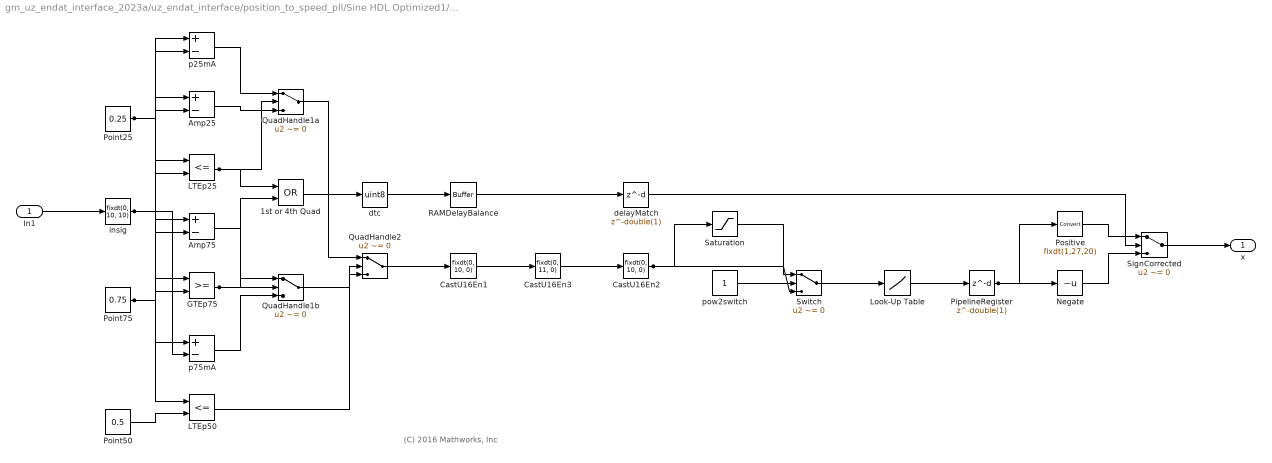
== system gm_uz_endat_interface_2023a/uz_endat_interface/position_to_speed_pll/Sine HDL Optimized1/sincos hdl/cos_hdl ==
  note: (C) 2016 Mathworks, Inc
  In1 : Inport  OutDataTypeStr=fixdt(1, 27, 20)  SampleTime=1e-08
  1st or 4th Quad : Logic  Operator=OR  AllPortsSameDT=off  OutDataTypeStr=boolean  SampleTime=1e-08
  Amp25 : Sum  Inputs=+-  AccumDataTypeStr=fixdt(1, 28, 27)  OutDataTypeStr=fixdt(1, 28, 27)  SampleTime=1e-08
  Amp75 : Sum  Inputs=+-  AccumDataTypeStr=fixdt(1, 28, 27)  OutDataTypeStr=fixdt(1, 28, 27)  SampleTime=1e-08
  CastU16En1 : DataTypeConversion  OutDataTypeStr=fixdt(0, 10, 0)  ConvertRealWorld=Stored Integer (SI)  SampleTime=1e-08  SaturateOnIntegerOverflow=off  RndMeth=Floor
  CastU16En2 : DataTypeConversion  OutDataTypeStr=fixdt(0, 10, 0)  ConvertRealWorld=Stored Integer (SI)  SampleTime=1e-08  RndMeth=Floor
  CastU16En3 : DataTypeConversion  OutDataTypeStr=fixdt(0, 11, 0)  SampleTime=1e-08  SaturateOnIntegerOverflow=off  RndMeth=Floor
  GTEp75 : RelationalOperator  OutDataTypeStr=boolean  SampleTime=1e-08  InputSameDT=off
  LTEp25 : RelationalOperator  Operator=<=  OutDataTypeStr=boolean  SampleTime=1e-08  InputSameDT=off
  LTEp50 : RelationalOperator  Operator=<=  OutDataTypeStr=boolean  SampleTime=1e-08  InputSameDT=off
  Look-Up Table : Lookup_n-D  NumberOfTableDimensions=1  BreakpointsForDimension1="fi(\"numerictype\",numerictype(0,10,0),\"fimath\",fimath(\"RoundingMethod\", \"Floor\",\"OverflowAction\", \"Wrap\",\"ProductMode\",\"FullPrecision\",\"SumMode\",\"FullPrecision\"),\"Value\",\"[0 1 2 3 4 5 6 7 8 9 10 11 12 13 14 15 16 17 18 19 20 21 22 23 24 25 26 27 28 29 30 31 32 33 34 35 36 37 38 39 40 41 42 43 44 45 46 47 48 49 50 51 52 53 54 55 56 57 58 59 60 61 62 63 64 65 66 67 68 69 70 71 72 73 74 75 76 77 78 79 80 81 82 83 84 85 86 87 88 89 90 91 92 93 94 95 96 97 98 99 100 101 102 103 104 105 106 107 108 109 110 111 112 113 114 115 116 117 118 119 120 121 122 123 124 125 126 127 128 129 130 131 132 133 134 135 136 137 138 139 140 141 142 143 144 145 146 147 148 149 150 151 152 153 154 155 156 157 158 159 160 161 162 163 164 165 166 167 168 169 170 171 172 173 174 175 176 177 178 179 180 181 182 183 184 185 186 187 188 189 190 191 192 193 194 195 196 197 198 199 200 201 202 203 204 205 206 207 208 209 210 211 212 213 214 215 216 217 218 219 220 221 222 223 224 225 226 227 228 229 230 231 232 233 234 235 236 237 238 239 240 241 242 243 244 245 246 247 248 249 250 251 252 253 254 255]\")"  Table="reshape(fi(\"numerictype\",numerictype(1,27,20),\"fimath\",fimath(\"RoundingMethod\", \"Floor\",\"OverflowAction\", \"Wrap\",\"ProductMode\",\"FullPrecision\",\"SumMode\",\"FullPrecision\"),\"Value\",\"[0;0.0061359405517578125;0.012271881103515625;0.01840686798095703125;0.02454090118408203125;0.03067493438720703125;0.03680706024169921875;0.042938232421875;0.04906749725341796875;0.055194854736328125;0.06132030487060546875;0.06744384765625;0.0735645294189453125;0.07968235015869140625;0.08579730987548828125;0.0919094085693359375;0.0980167388916015625;0.10412120819091796875;0.11022186279296875;0.11631870269775390625;0.12241077423095703125;0.128498077392578125;0.1345806121826171875;0.14065837860107421875;0.1467304229736328125;0.15279674530029296875;0.15885829925537109375;0.164913177490234375;0.17096233367919921875;0.1770038604736328125;0.18303966522216796875;0.18906879425048828125;0.19509029388427734375;0.20110416412353515625;0.207111358642578125;0.2131099700927734375;0.2191009521484375;0.2250843048095703125;0.2310581207275390625;0.23702335357666015625;0.24298000335693359375;0.248928070068359375;0.2548656463623046875;0.2607936859130859375;0.26671314239501953125;0.27262115478515625;0.27851963043212890625;0.28440761566162109375;0.2902851104736328125;0.29615116119384765625;0.302005767822265625;0.307849884033203125;0.31368160247802734375;0.3195018768310546875;0.32531070709228515625;0.3311061859130859375;0.33689022064208984375;0.3426609039306640625;0.34841823577880859375;0.35416316986083984375;0.35989475250244140625;0.36561298370361328125;0.3713169097900390625;0.37700748443603515625;0.38268375396728515625;0.38834476470947265625;0.39399242401123046875;0.399623870849609375;0.4052410125732421875;0.4108428955078125;0.4164295196533203125;0.42199993133544921875;0.427555084228515625;0.433094024658203125;0.4386157989501953125;0.444122314453125;0.449611663818359375;0.4550838470458984375;0.4605388641357421875;0.465976715087890625;0.47139644622802734375;0.47679901123046875;0.4821834564208984375;0.48754978179931640625;0.49289798736572265625;0.4982280731201171875;0.5035381317138671875;0.50883007049560546875;0.514102935791015625;0.51935577392578125;0.52458953857421875;0.52980327606201171875;0.5349979400634765625;0.54017162322998046875;0.54532527923583984375;0.55045795440673828125;0.5555706024169921875;0.56066131591796875;0.56573200225830078125;0.57078075408935546875;0.57580852508544921875;0.580814361572265625;0.5857982635498046875;0.59075927734375;0.595699310302734375;0.600616455078125;0.605510711669921875;0.61038303375244140625;0.61523151397705078125;0.62005710601806640625;0.62485980987548828125;0.629638671875;0.6343936920166015625;0.63912487030029296875;0.6438312530517578125;0.64851474761962890625;0.65317249298095703125;0.657806396484375;0.66241550445556640625;0.66699981689453125;0.67155933380126953125;0.67609310150146484375;0.6806011199951171875;0.6850833892822265625;0.689540863037109375;0.6939716339111328125;0.69837665557861328125;0.702754974365234375;0.70710659027099609375;0.71143245697021484375;0.7157306671142578125;0.72000217437744140625;0.724246978759765625;0.7284641265869140625;0.732654571533203125;0.73681640625;0.7409515380859375;0.7450580596923828125;0.7491359710693359375;0.7531871795654296875;0.75720882415771484375;0.76120281219482421875;0.765167236328125;0.76910305023193359375;0.77301025390625;0.77688884735107421875;0.7807369232177734375;0.78455638885498046875;0.78834629058837890625;0.79210662841796875;0.79583644866943359375;0.79953765869140625;0.8032073974609375;0.80684757232666015625;0.8104572296142578125;0.81403636932373046875;0.817584991455078125;0.821102142333984375;0.82458972930908203125;0.828044891357421875;0.83146953582763671875;0.83486270904541015625;0.8382244110107421875;0.8415546417236328125;0.84485340118408203125;0.84812068939208984375;0.85135555267333984375;0.85455799102783203125;0.8577289581298828125;0.860866546630859375;0.86397266387939453125;0.867046356201171875;0.870086669921875;0.8730945587158203125;0.8760700225830078125;0.87901210784912109375;0.88192081451416015625;0.88479709625244140625;0.8876399993896484375;0.89044857025146484375;0.8932247161865234375;0.89596652984619140625;0.89867401123046875 ...(+1615 chars)]\"), [1  256])"  InterpMethod=Flat  ExtrapMethod=Clip  DiagnosticForOutOfRangeInput=Error  SampleTime=1e-08  OutDataTypeStr=fixdt(1, 27, 20)
  Negate : UnaryMinus  SampleTime=1e-08
  PipelineRegister : Delay  DelayLength=double(1)  InitialCondition=0
  Point25 : Constant  Value=0.25  OutDataTypeStr=fixdt(0, 27, 27)  SampleTime=1e-08
  Point50 : Constant  Value=0.5  OutDataTypeStr=fixdt(0, 27, 27)  SampleTime=1e-08
  Point75 : Constant  Value=0.75  OutDataTypeStr=fixdt(0, 27, 27)  SampleTime=1e-08
  Positive : DataTypeConversion  OutDataTypeStr=fixdt(1,27,20)
  QuadHandle1a : Switch  Criteria=u2 ~= 0  Threshold=double(0)  OutDataTypeStr=fixdt(1, 28, 27)  SampleTime=1e-08  SaturateOnIntegerOverflow=off  InputSameDT=off
  QuadHandle1b : Switch  Criteria=u2 ~= 0  Threshold=double(0)  OutDataTypeStr=fixdt(1, 28, 27)  SampleTime=1e-08  SaturateOnIntegerOverflow=off  InputSameDT=off
  QuadHandle2 : Switch  Criteria=u2 ~= 0  Threshold=double(0)  OutDataTypeStr=fixdt(0, 10, 10)  SampleTime=1e-08  InputSameDT=off
  RAMDelayBalance : hdlmdlgenlib/Buffer
  Saturation : Saturate  UpperLimit="fi(0,0,10,0,\"hex\",\"0ff\")"  LowerLimit="fi(0,0,10,0,\"hex\",\"000\")"  SampleTime=1e-08  OutDataTypeStr=fixdt(0, 10, 0)
  SignCorrected : Switch  Criteria=u2 ~= 0  Threshold=double(0)  OutDataTypeStr=fixdt(1, 27, 20)  SampleTime=1e-08  SaturateOnIntegerOverflow=off  InputSameDT=off
  Switch : Switch  Criteria=u2 ~= 0  Threshold=double(0)  OutDataTypeStr=fixdt(0, 10, 0)  SampleTime=1e-08  SaturateOnIntegerOverflow=off  InputSameDT=off
  delayMatch : Delay  DelayLength=double(1)  InitialCondition=0
  dtc : DataTypeConversion  OutDataTypeStr=uint8  ConvertRealWorld=Stored Integer (SI)  SampleTime=1e-08  SaturateOnIntegerOverflow=off  RndMeth=Floor
  insig : DataTypeConversion  OutDataTypeStr=fixdt(0, 10, 10)  SampleTime=1e-08  SaturateOnIntegerOverflow=off  RndMeth=Floor
  p25mA : Sum  Inputs=+-  AccumDataTypeStr=fixdt(1, 28, 27)  OutDataTypeStr=fixdt(1, 28, 27)  SampleTime=1e-08
  p75mA : Sum  Inputs=+-  AccumDataTypeStr=fixdt(1, 28, 27)  OutDataTypeStr=fixdt(1, 28, 27)  SampleTime=1e-08
  pow2switch : Constant  OutDataTypeStr=boolean  SampleTime=1e-08
  x : Outport  SampleTime=1e-08  InitialOutput=0
  wires:
  dtc/1 -> RAMDelayBalance/1
  Amp25/1 -> QuadHandle1a/3
  Amp75/1 -> QuadHandle1b/1
  CastU16En1/1 -> CastU16En3/1
  CastU16En2/1 -> Switch/3, Saturation/1
  CastU16En3/1 -> CastU16En2/1
  GTEp75/1 -> QuadHandle1b/2, 1st or 4th Quad/2
  LTEp25/1 -> QuadHandle1a/2, 1st or 4th Quad/1
  LTEp50/1 -> QuadHandle2/2
  PipelineRegister/1 -> Positive/1, Negate/1
  Negate/1 -> SignCorrected/3
  Point25/1 -> p25mA/1, LTEp25/2, Amp25/2
  Point50/1 -> LTEp50/2
  Point75/1 -> p75mA/1, GTEp75/2, Amp75/2
  Positive/1 -> SignCorrected/1
  QuadHandle1a/1 -> QuadHandle2/1
  QuadHandle1b/1 -> QuadHandle2/3
  QuadHandle2/1 -> CastU16En1/1
  delayMatch/1 -> SignCorrected/2
  Saturation/1 -> Switch/1
  SignCorrected/1 -> x/1
  Switch/1 -> Look-Up Table/1
  insig/1 -> p75mA/2, p25mA/2, LTEp50/1, LTEp25/1, GTEp75/1, Amp75/1, Amp25/1
  p25mA/1 -> QuadHandle1a/1
  p75mA/1 -> QuadHandle1b/3
  pow2switch/1 -> Switch/2
  1st or 4th Quad/1 -> dtc/1
  In1/1 -> insig/1
  RAMDelayBalance/1 -> delayMatch/1
  Look-Up Table/1 -> PipelineRegister/1
